simulink subsystem "HO_AnalogOutputs"  (R2019b)
settings: Solver=VariableStepAuto  StartTime=0.0  StopTime=10.0  RelTol=1e-3
undefined symbols (not defined in the file): Down, GPTRIP1SEL, GPTRIP2SEL, motorPWMFreq, TZ1, TZ2, Up
libraries: FunctionCallDivider x1, c2837xDlib x1, c2802xlib x1
settings Model: Creator=Nick  LastModifiedBy=Nick

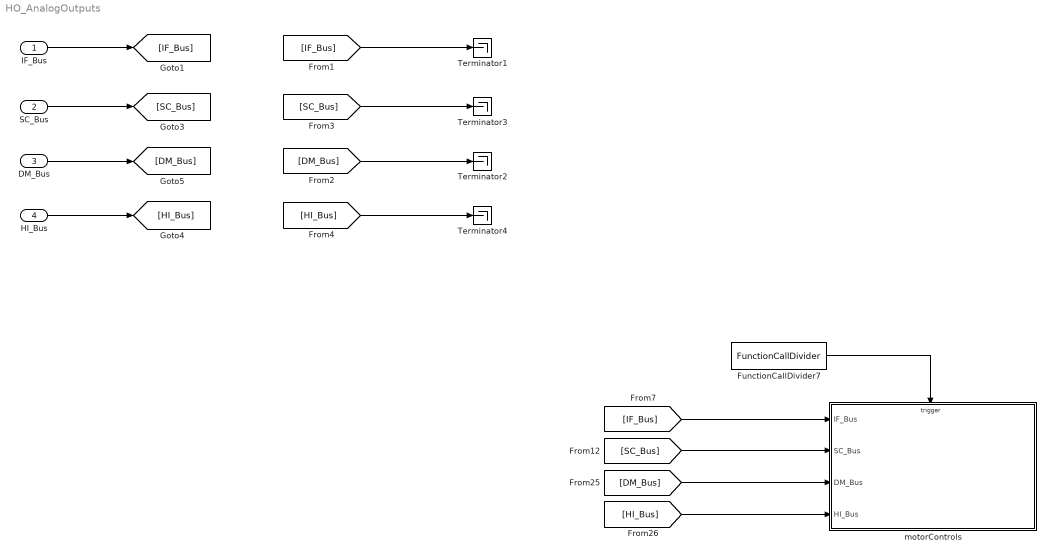
== system HO_AnalogOutputs ==
  IF_Bus : Inport
  SC_Bus : Inport  Port=2
  DM_Bus : Inport  Port=3
  HI_Bus : Inport  Port=4
  FunctionCallDivider7 : FunctionCallDivider/Algroithms/FunctionCallDivider  counts=1
  Terminator{1..4} (4 alike) : Terminator
  motorControls : Subsystem  TreatAsAtomicUnit=on
  wires:
  [IF_Bus] -> Terminator1/1
  [DM_Bus] -> Terminator2/1
  [SC_Bus] -> Terminator3/1
  DM_Bus/1 -> [DM_Bus]
  SC_Bus/1 -> [SC_Bus]
  HI_Bus/1 -> [HI_Bus]
  [HI_Bus] -> Terminator4/1
  IF_Bus/1 -> [IF_Bus]
  [HI_Bus] -> motorControls/4(HI_Bus)
  [DM_Bus] -> motorControls/3(DM_Bus)
  [IF_Bus] -> motorControls/1(IF_Bus)
  [SC_Bus] -> motorControls/2(SC_Bus)
  FunctionCallDivider7/1 -> motorControls/Trigger

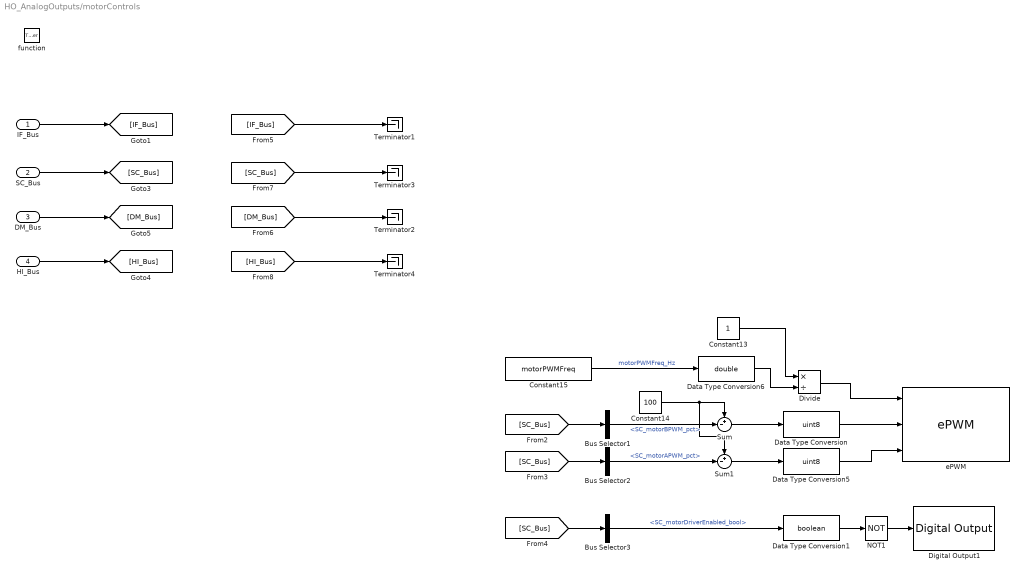
== system HO_AnalogOutputs/motorControls ==
  IF_Bus : Inport
  SC_Bus : Inport  Port=2
  DM_Bus : Inport  Port=3
  HI_Bus : Inport  Port=4
  function : TriggerPort  TriggerType=function-call  VariantControl=Variant
  Bus Selector1 : BusSelector  OutputSignals=motorControlBus.SC_motorBPWM_pct
  Bus Selector2 : BusSelector  OutputSignals=motorControlBus.SC_motorAPWM_pct
  Bus Selector3 : BusSelector  OutputSignals=motorControlBus.SC_motorDriverEnabled_bool
  Constant13 : Constant
  Constant14 : Constant  Value=100
  Constant15 : Constant  Value=motorPWMFreq
  Data Type Conversion : DataTypeConversion  OutDataTypeStr=uint8
  Data Type Conversion1 : DataTypeConversion  OutDataTypeStr=boolean
  Data Type Conversion5 : DataTypeConversion  OutDataTypeStr=uint8
  Data Type Conversion6 : DataTypeConversion  OutDataTypeStr=double
  Digital Output1 : c2837xDlib/Digital Output  GPIO_Number=GPIO16~GPIO23  GPIO_Bit0=on  GPIO_BIT0_Toggle=off  GPIO_Bit1=off  GPIO_BIT1_Toggle=off  GPIO_Bit2=off  GPIO_BIT2_Toggle=off  GPIO_Bit3=off  GPIO_BIT3_Toggle=off  GPIO_Bit4=off  GPIO_BIT4_Toggle=off  GPIO_Bit5=off  GPIO_BIT5_Toggle=off  GPIO_Bit6=off  GPIO_BIT6_Toggle=off  GPIO_Bit7=off  GPIO_BIT7_Toggle=off
      settings: SourceProductName=Embedded Coder Support Package for Texas Instruments C2000 Processors  SourceProductBaseCode=TIC2000
  Divide : Product  Inputs=*/
  NOT1 : Logic  Operator=NOT  IconShape=distinctive  AllPortsSameDT=off  OutDataTypeStr=boolean
  Sum : Sum  Inputs=+-|
  Sum1 : Sum  Inputs=+-|
  Terminator{1..4} (4 alike) : Terminator
  ePWM : c2802xlib/ePWM  useModule=ePWM2  ePWMxLINKTBPRD=Not Linked  periodUnits=Seconds  timerSource=Input port  timerPeriod_clk=64000  timerPeriod_sec=0.0001  tbshadow=Counter equals to zero  countingMode=Up-Down  phaseActiveEnable=Disable  phaseDirection=Count down after sync  phaseActive=0  synchronizationEnable=off  dcaevt1Sync=off  dcbevt1Sync=off  synchronizationOption=Disable  clockPrescale=1  HSclockPrescale=1  enswap=off  ePWMxAStatus=on  ePWMxAactionLogic1=Set  ePWMxAactionLogic2=Clear  ePWMxAactionLogic3=Clear  ePWMxAactionLogic4=Set  ePWMxAactionLogic5=Do nothing  ePWMxAactionLogic6=Do nothing  ePWMxALoadMode=Load on counter equals to zero (CTR=Zero)  ePWMxACSFenable=off  ePWMxACSFvalue=Forcing disable  ePWMxASFreload=Zero  ePWMxBStatus=on  ePWMxBactionLogic1=Set  ePWMxBactionLogic2=Clear  ePWMxBactionLogic3=Do nothing  ePWMxBactionLogic4=Do nothing  ePWMxBactionLogic5=Clear  ePWMxBactionLogic6=Set  ePWMxBLoadMode=Load on counter equals to zero (CTR=Zero)  ePWMxBCSFenable=off  ePWMxBCSFvalue=Forcing disable  ePWMxBSFreload=Zero  ePWNxBOutWay=off  ePWMxLINKCMPA=Not Linked  CMPAUnits=Percentages  CMPASource=Input port  CMPAValue_per=0  CMPAValue_clk=32000  enCMPAshadow=Counter equals to zero  ePWMxLINKCMPB=Not Linked  CMPBUnits=Percentages  CMPBSource=Input port  CMPBValue_per=0  CMPBValue_clk=32000  enCMPBshadow=Counter equals to zero  ePWMxLINKCMPC=Not Linked  CMPCUnits=Clock cycles  CMPCSource=Specify via dialog  CMPCValue_per=50  CMPCValue_clk=32000  enCMPCshadow=Counter equals to zero  ePWMxLINKCMPD=Not Linked  CMPDUnits=Clock cycles  CMPDSource=Specify via dialog  CMPDValue_per=50  CMPDValue_clk=32000  enCMPDshadow=Counter equals to zero  enableDBePWMxA=off  enableDBePWMxB=off  enhalfcycle=off  DBpolarity=Active high (AH)  DBedgeDelay=Positive  DBSource_ePWMxA=ePWMxA  DBSource_ePWMxB=ePWMxA  DBperiodSource=Specify via dialog  REDperiod=0  FEDperiod=0  adcstartModuleA=off  adcrequestEventA=First event  adcstartEventA=Digital Compare Module A Event 1 start of conversion (DCAEVT1.soc)  adcstartEventA_type2=Digital Compare Module A Event 1 start of conversion (DCAEVT1.soc)  adcstartModuleB=off  adcrequestEventB=First event  adcstartEventB=Counter equals to zero (CTR=Zero)  adcstartEventB_type2=Counter equals to zero (CTR=Zero)  intEn=off  intPrd=First event  intSel=Counter equals to zero (CTR=Zero)  intSel_type2=Counter equals to zero (CTR=Zero)  hrpe=off  enHRPWM=off  HRPWM_LoadMode=Counter equals to period (CTR=PRD)  HRPWM_CTLMode=Duty or Period control mode  HRPWM_EDGMode=Both edge  hrpeb=off  enHRPWMB=off  HRPWM_LoadModeB=Counter equals to zero (CTR=ZERO)  HRPWM_CTLModeB=Duty or Period control mode  HRPWM_EDGModeB=Both edge  enSFO=on  enautoconv=on  chopperEnable=off  chopperFrequency=1  chopperFirstwidth=1  chopperDuty=12.5%  tripZonesource=Specify via dialog  tzselOSHT1=off  tzselOSHT2=off  tzselOSHT3=off  tzselOSHDCAEV1=off  tzselOSHDCBEV1=off  tzselCBC1=off  tzselCBC2=off  tzselCBC3=off  tzselCBCDCAEV2=off  tzselCBCDCBEV2=off  tzselOSHT4=off  tzselOSHT5=off  tzselOSHT6=off  tzselCBC4=off  tzselCBC5=off  tzselCBC6=off  enTzOstIntr=off  enTzCbcIntr=off  enTzDCAEVT1Intr=off  enTzDCAEVT2Intr=off  enTzDCBEVT1Intr=off  enTzDCBEVT2Intr=off  ePWMxAforced=No action  ePWMxBforced=No action  DCAEVT1forced=No action  DCBEVT1forced=No action  DCAEVT2forced=No action  DCBEVT2forced=No action  dcah=Trip Zone 1 input (TZ1)  dcal=Trip Zone 2 input (TZ2)  dcbh=Trip Zone 1 input (TZ1)  dcbl=Trip Zone 2 input (TZ2)  dcah_type2=GPTRIP1SEL/(TZ1)  dcal_type2=GPTRIP2SEL/(TZ2)  dcbh_type2=GPTRIP1SEL/(TZ1)  dcbl_type2=GPTRIP2SEL/(TZ2)  gendcaevt1=Event disabled  gendcaevt2=Event disabled  gendcbevt1=Event disabled  gendcbevt2=Event disabled  dcaevt1src=DCAEVT1 with sync  dcaevt2src=DCAEVT2 with sync  dcbevt1src=DCBEVT1 with sync  dcbevt2src=DCBEVT2 with sync  pulsesel=Counter equals to zero (CTR=Zero)  blankinv=off  blankoffset=0  blankwidth=0  evsrcsel=Filtered version of DCAEVT1 (DCAEVT1FILT)  encape=off  PwmType=C2000_Type4
      settings: SourceProductName=Embedded Coder Support Package for Texas Instruments C2000 Processors
  wires:
  NOT1/1 -> Digital Output1/1
  Data Type Conversion1/1 -> NOT1/1
  Constant15/1 -> Data Type Conversion6/1  "motorPWMFreq_Hz"
  Data Type Conversion/1 -> ePWM/2
  Constant13/1 -> Divide/1
  Divide/1 -> ePWM/1
  Constant14/1 -> Sum1/1, Sum/1
  Sum/1 -> Data Type Conversion/1
  Data Type Conversion6/1 -> Divide/2
  Sum1/1 -> Data Type Conversion5/1
  Data Type Conversion5/1 -> ePWM/3
  Bus Selector2/1 -> Sum1/2  "<SC_motorAPWM_pct>"
  Bus Selector1/1 -> Sum/2  "<SC_motorBPWM_pct>"
  [SC_Bus] -> Bus Selector1/1
  [SC_Bus] -> Bus Selector2/1
  [SC_Bus] -> Bus Selector3/1
  Bus Selector3/1 -> Data Type Conversion1/1  "<SC_motorDriverEnabled_bool>"
  [IF_Bus] -> Terminator1/1
  [DM_Bus] -> Terminator2/1
  [SC_Bus] -> Terminator3/1
  DM_Bus/1 -> [DM_Bus]
  SC_Bus/1 -> [SC_Bus]
  HI_Bus/1 -> [HI_Bus]
  [HI_Bus] -> Terminator4/1
  IF_Bus/1 -> [IF_Bus]
